simulink model "CHM2ActiveReqChk"  (R2018b)
settings: Solver=FixedStepDiscrete  StartTime=0.0  StopTime=10.0  RelTol=1e-3
libraries: simulink x2
settings Model: Creator=sn2xws  LastModifiedBy=sn2xws
settings DataIOCC: SaveFormat=StructureWithTime
settings OptimizationCC: DefaultParameterBehavior=Inlined  EnhancedBackFolding=on  PassReuseOutputArgsAs=Individual arguments  ZeroExternalMemoryAtStartup=off  ZeroInternalMemoryAtStartup=off  OptimizeBlockOrder=speed  DifferentSizesBufferReuse=on  OptimizationCustomize=off
settings DebuggingCC: ParameterTunabilityLossMsg=error
settings SFSimCC: MATLABDynamicMemAlloc=off
settings RTWCC: SystemTargetFile=autosar.tlc  GenCodeOnly=on  TemplateMakefile=ert_default_tmf  Description=AUTOSAR  GenerateReport=on  IncludeHyperlinkInReport=on  LaunchReport=on  GenerateTraceInfo=on  GenerateTraceReport=on  GenerateTraceReportSl=on  GenerateTraceReportSf=on  GenerateTraceReportEml=on
settings CodeAppCC: ForceParamTrailComments=on  IgnoreCustomStorageClasses=off  OperatorAnnotations=on  SimulinkDataObjDesc=on  SFDataObjDesc=on  InsertBlockDesc=on
settings STFCustomTargetCC: TargetLangStandard=C99 (ISO)  MultiwordLength=256  ParMdlRefBuildCompliant=on  CompOptLevelCompliant=on  IncludeMdlTerminateFcn=off  CombineOutputUpdateFcns=on  SuppressErrorStatus=on  ERTCustomFileBanners=on  SupportNonFinite=off  SupportComplex=off  SupportContinuousTime=off  SupportNonInlinedSFcns=off  RemoveResetFunc=on  MATLABClassNameForMDSCustomization=Simulink.SoftwareTarget.ERTCustomization  AutosarCompliant=on  UseToolchainInfoCompliant=on  LookupTableObjectStructAxisOrder=2,1,3,4,...  LUTObjectStructOrderEvenSpacing=Size,Table,Breakpoints  SystemTargetFile=autosar.tlc
settings ERTTargetCC: TargetLangStandard=C99 (ISO)  ConcurrentExecutionCompliant=off  IncludeMdlTerminateFcn=off  SuppressErrorStatus=on  SupportNonFinite=off  SupportComplex=off  ModelStepFunctionPrototypeControlCompliant=off  CPPClassGenCompliant=off  AutosarCompliant=on  LookupTableObjectStructAxisOrder=2,1,3,4,...  LUTObjectStructOrderEvenSpacing=Size,Table,Breakpoints  InlinedParameterPlacement=NonHierarchical  ERTCustomFileTemplate=example_file_process.tlc  ERTFilePackagingFormat=Compact

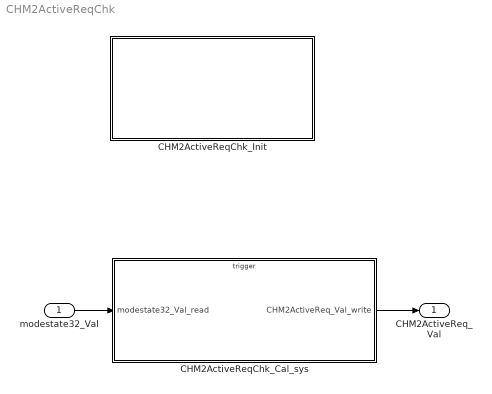
== system CHM2ActiveReqChk ==
  modestate32_Val : Inport  OutDataTypeStr=uint32  PortDimensions=1
  CHM2ActiveReqChk_Cal_sys : Subsystem
  CHM2ActiveReqChk_Init : Subsystem
  CHM2ActiveReq_Val : Outport  OutDataTypeStr=boolean  PortDimensions=1
  wires:
  modestate32_Val/1 -> CHM2ActiveReqChk_Cal_sys/1(modestate32_Val_read)
  CHM2ActiveReqChk_Cal_sys/1(CHM2ActiveReq_Val_write) -> CHM2ActiveReq_Val/1

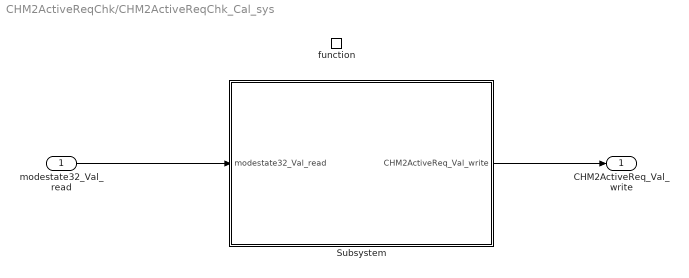
== system CHM2ActiveReqChk/CHM2ActiveReqChk_Cal_sys ==
  modestate32_Val_read : Inport
  function : TriggerPort  TriggerType=function-call  IsSimulinkFunction=on  FunctionName=CHM2ActiveReqChk_Cal  VariantControl=(inherit)
  Subsystem : Subsystem
  CHM2ActiveReq_Val_write : Outport
      settings: EnsureOutportIsVirtual=on
  wires:
  modestate32_Val_read/1 -> Subsystem/1(modestate32_Val_read)
  Subsystem/1(CHM2ActiveReq_Val_write) -> CHM2ActiveReq_Val_write/1

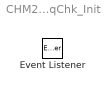
== system CHM2ActiveReqChk/CHM2ActiveReqChk_Init ==
  Event Listener : EventListener  EventName=reset

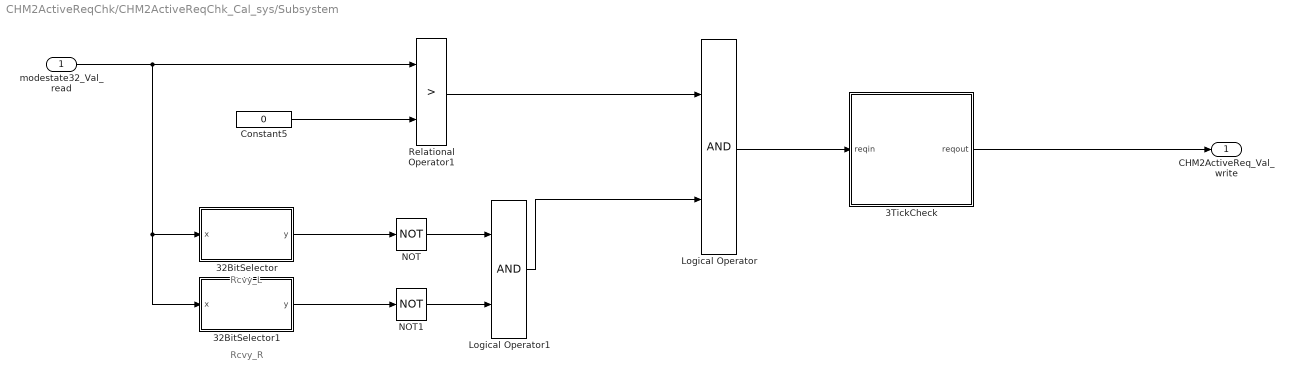
== system CHM2ActiveReqChk/CHM2ActiveReqChk_Cal_sys/Subsystem ==
  note: Rcvy_R
  note: Rcvy_L
  modestate32_Val_read : Inport
  32BitSelector : Subsystem  mask(32 Bit Selector){BitNum=10}
      mask prompts: BitNum "Select Bit Number"
      mask help: Allows selection of a particular bit (0-31) out of a packed word up to 32 bits long. Output will be true if the bit number selected via the mask parameter is equal to one.
      mask TypeOptions BitNum: 0 | 1 | 2 | 3 | 4 | 5 | 6 | 7 | 8 | 9 | 10 | 11 | 12 | 13 | 14 | 15 | 16 | 17 | 18 | 19 | 20 | 21 | 22 | 23 | 24 | 25 | 26 | 27 | 28 | 29 | 30 | 31
      mask Display:
      | text(0.5, 0.8,'BIT','horizontalAlignment','center')
      | text(0.5, 0.5,'SELECTOR','horizontalAlignment','center')
      | text(0.5, 0.2,['-- Bit ',char(get_param(gcb,'BitNum')),' --'],'horizontalAlignment','center')
  32BitSelector1 : Subsystem  mask(32 Bit Selector){BitNum=12}
      mask prompts: BitNum "Select Bit Number"
      mask help: Allows selection of a particular bit (0-31) out of a packed word up to 32 bits long. Output will be true if the bit number selected via the mask parameter is equal to one.
      mask TypeOptions BitNum: 0 | 1 | 2 | 3 | 4 | 5 | 6 | 7 | 8 | 9 | 10 | 11 | 12 | 13 | 14 | 15 | 16 | 17 | 18 | 19 | 20 | 21 | 22 | 23 | 24 | 25 | 26 | 27 | 28 | 29 | 30 | 31
      mask Display:
      | text(0.5, 0.8,'BIT','horizontalAlignment','center')
      | text(0.5, 0.5,'SELECTOR','horizontalAlignment','center')
      | text(0.5, 0.2,['-- Bit ',char(get_param(gcb,'BitNum')),' --'],'horizontalAlignment','center')
  3TickCheck : Subsystem
  Constant5 : Constant  Value=0  OutDataTypeStr=uint32
  Logical Operator : Logic  AllPortsSameDT=off  OutDataTypeStr=boolean
  Logical Operator1 : Logic  AllPortsSameDT=off  OutDataTypeStr=boolean
  NOT : Logic  Operator=NOT  AllPortsSameDT=off  OutDataTypeStr=boolean
  NOT1 : Logic  Operator=NOT  AllPortsSameDT=off  OutDataTypeStr=boolean
  Relational Operator1 : RelationalOperator  Operator=>  OutDataTypeStr=boolean  RndMeth=Simplest
  CHM2ActiveReq_Val_write : Outport
      settings: EnsureOutportIsVirtual=on
  wires:
  3TickCheck/1(reqout) -> CHM2ActiveReq_Val_write/1
  modestate32_Val_read/1 -> 32BitSelector/1(x), 32BitSelector1/1(x), Relational Operator1/1
  Logical Operator1/1 -> Logical Operator/2
  NOT/1 -> Logical Operator1/1
  32BitSelector1/1(y) -> NOT1/1
  Relational Operator1/1 -> Logical Operator/1
  Logical Operator/1 -> 3TickCheck/1(reqin)
  Constant5/1 -> Relational Operator1/2
  32BitSelector/1(y) -> NOT/1
  NOT1/1 -> Logical Operator1/2

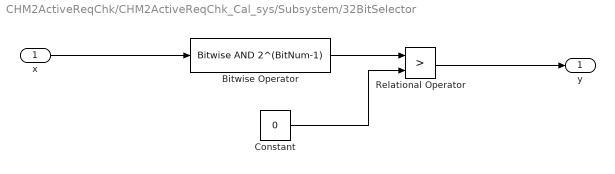
== system CHM2ActiveReqChk/CHM2ActiveReqChk_Cal_sys/Subsystem/32BitSelector ==
  x : Inport
  Bitwise Operator : simulink/Logic and Bit Operations/Bitwise Operator  logicop=AND  UseBitMask=on  BitMask=2^(BitNum-1)  BitMaskRealWorld=Stored Integer
  Constant : Constant  Value=0  OutDataTypeStr=uint32
  Relational Operator : RelationalOperator  Operator=>  OutDataTypeStr=boolean  RndMeth=Simplest
  y : Outport
  wires:
  Bitwise Operator/1 -> Relational Operator/1
  x/1 -> Bitwise Operator/1
  Constant/1 -> Relational Operator/2
  Relational Operator/1 -> y/1

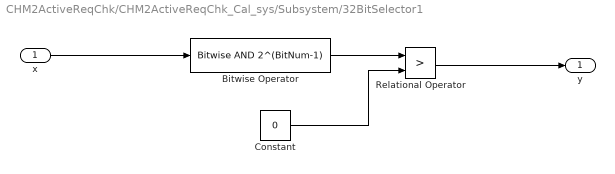
== system CHM2ActiveReqChk/CHM2ActiveReqChk_Cal_sys/Subsystem/32BitSelector1 ==
  x : Inport
  Bitwise Operator : simulink/Logic and Bit Operations/Bitwise Operator  logicop=AND  UseBitMask=on  BitMask=2^(BitNum-1)  BitMaskRealWorld=Stored Integer
  Constant : Constant  Value=0  OutDataTypeStr=uint32
  Relational Operator : RelationalOperator  Operator=>  OutDataTypeStr=boolean  RndMeth=Simplest
  y : Outport
  wires:
  Bitwise Operator/1 -> Relational Operator/1
  x/1 -> Bitwise Operator/1
  Constant/1 -> Relational Operator/2
  Relational Operator/1 -> y/1

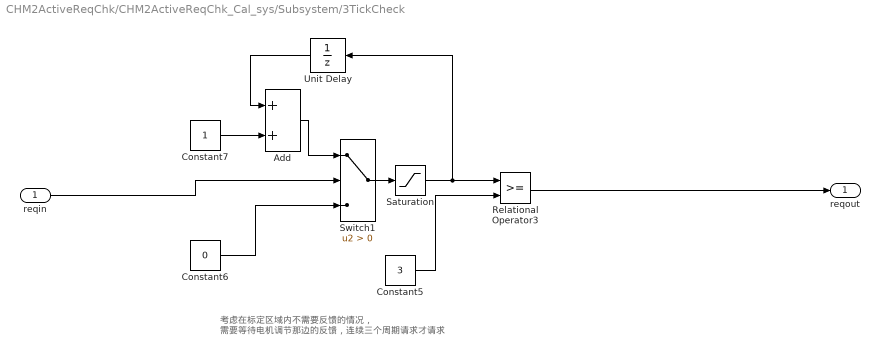
== system CHM2ActiveReqChk/CHM2ActiveReqChk_Cal_sys/Subsystem/3TickCheck ==
  note: 考虑在标定区域内不需要反馈的情况，
      | 需要等待电机调节那边的反馈，连续三个周期请求才请求
  reqin : Inport
  Add : Sum
  Constant5 : Constant  Value=3  OutDataTypeStr=uint8
  Constant6 : Constant  Value=0  OutDataTypeStr=uint8
  Constant7 : Constant  OutDataTypeStr=uint8
  Relational Operator3 : RelationalOperator  OutDataTypeStr=boolean  RndMeth=Simplest
  Saturation : Saturate  UpperLimit=3  LowerLimit=0  OutDataTypeStr=uint8
  Switch1 : Switch  Criteria=u2 > Threshold
  Unit Delay : UnitDelay  SampleTime=-1
  reqout : Outport
  wires:
  Relational Operator3/1 -> reqout/1
  reqin/1 -> Switch1/2
  Switch1/1 -> Saturation/1
  Add/1 -> Switch1/1
  Saturation/1 -> Relational Operator3/1, Unit Delay/1
  Constant7/1 -> Add/2
  Constant5/1 -> Relational Operator3/2
  Constant6/1 -> Switch1/3
  Unit Delay/1 -> Add/1
